simulink model "Imitation_Task_Multi_withSound_withGrid"  (R2015a)
settings: Solver=ode4  SolverMode=MultiTasking  StartTime=0.0  StopTime=inf  FixedStep=BKIN_STEP_TIME  RelTol=1e-3
StartFcn:
  |  warndlg('Dexterit-E models cannot run under simulation. Please compile your model and run it from within Dexterit-E.');set_param(bdroot,'SimulationCommand','stop')
model workspace (MAT data in the model file):
  col_x = 1
  col_y = 2
  RADIUS_VIS = 3
  COLOR_INIT = 4
  START_TARGET_COL = 1
  DELAY_POST_TRIAL_COL = 20
  BKIN_STEP_TIME = 0.00025
  COLOR_MOVE = 5
  START_WAIT_TIME_COL = 2
  CUE_TARGET_COL = 3
  STIM_DUR_COL = 17
  MAX_MOVE_TIME_COL = 18
  HOLD_TIME_COL = 19
  E_START_TRIAL = 2
  E_START_REACHED = 4
  E_MOVED_EARLY = 21
  E_GO_CUE = 9
  E_MOVE_TIMEOUT = 23
  E_HOLDING_STILL = 12
  E_END_TRIAL = 14
  CONTROL_PT1_COL = 8
  CONTROL_PT2_COL = 9
  CONTROL_PT3_COL = 10
  CONTROL_PT4_COL = 11
  STROKE_WIDTH = 6
  K_HAND_VEL = 1
  E_MOVE_ON = 10
  CUE_TYPE_COL = 6
  CUE_VIS_COL = 4
  HAND_VIS_COL = 5
  K_HOLDTIME = 2
  K_ROBOT_RAMP_TIME = 3
  E_ROBOT_RETURN_TO_START = 33
  E_ENABLED_CONTROLLER = 31
  K_TIME_TO_START = 4
  E_RETURN_TO_START = 35
  E_HOLD_POS = 37
  CONTROL_PT5_COL = 12
  CONTROL_PT6_COL = 13
  CONTROL_PT7_COL = 14
  CONTROL_PT8_COL = 15
  CONTROL_PT9_COL = 16
  E_INCREMENTING_TSTEP1 = 6
  E_INCREMENTING_TSTEP2 = 7
  E_INCREMENTING_TSTEP3 = 8
  CONTROL_PT0_COL = 7
  K_TONE_START_FREQUENCY = 5
  K_TONE_START_DURATION = 6
  K_TONE_GO_FREQUENCY = 7
  K_TONE_GO_DURATION = 8
  ENABLE_BKGND_GRID_COL = 21
  BKGND_GRID_TGT_COL = 22
  BKIN_KINEMATIC_FRAME_SIZE = 400
  E_NO_EVENT = 0
libraries: slrtlib x9, Video x7, General x3, KINARM_general x2, KINARM_loads x2, xpcobsoletelib x1, xpcrtudplib x1
CloseFcn:
  | rtwprivate ssgencode ModelCloseRequest b2lab2d
settings Model: ModifiedComment=chris -- Wed Feb 16 09:18:30 2005 -- Version 1.1384  ModifiedHistory=Feb 16/05 - Add error repeat, add offset ramp  ExtModeArmWhenConnect=off  ExtModeLogAll=off  Creator=Chris Grebeldinger  LastModifiedBy=User
settings SolverCC: EnableConcurrentExecution=on  AutoInsertRateTranBlk=on
settings DataIOCC: LimitDataPoints=off  SignalLoggingSaveFormat=ModelDataLogs  SaveOutput=off  SaveTime=off  SignalLoggingName=sigsOut
settings OptimizationCC: BlockReduction=off  BooleanDataType=off  OptimizeBlockIOStorage=off  BufferReuse=off  GlobalBufferReuse=off  ExpressionFolding=off  ExpressionDepthLimit=2147483647  LocalBlockOutputs=off  InitFltsAndDblsToZero=on
settings DebuggingCC: SaveWithParameterizedLinksMsg=none  UnderspecifiedInitializationDetection=Classic  MergeDetectMultiDrivingBlocksExec=none  SignalResolutionControl=TryResolveAllWithWarning  MultiTaskDSMMsg=warning  FcnCallInpInsideContextMsg=UseLocalSettings  StateNameClashWarn=warning  StrictBusMsg=ErrorOnBusTreatedAsVector
settings HardwareCC: ProdIntDivRoundTo=Zero  ProdEndianess=LittleEndian  ProdLongLongMode=on  ProdHWDeviceType=Generic->32-bit x86 compatible  TargetHWDeviceType=32-bit Generic
settings SFSimCC: SimCustomHeaderCode="#include \"stdlib.h\""  SFSimEcho=off  SimParseCustomCode=off
settings RTWCC: SystemTargetFile=slrt.tlc  TemplateMakefile=slrt_default_tmf  Description=Simulink Real-Time  CustomSourceCode="#include \"stdlib.h\""
settings CodeAppCC: MaxIdLength=63
settings SimulinkRealTimeCC: TargetFcnLib=ansi_tfl_tmw.mat  GeneratePreprocessorConditionals=Disable all  xPCisDownloadable=off  xPCisDefaultEnv=off

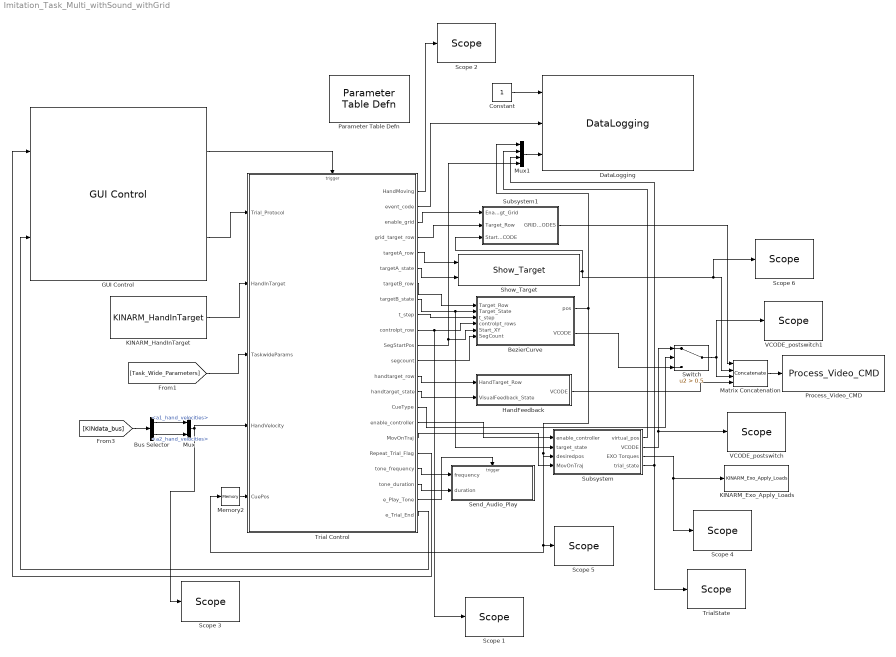
== system Imitation_Task_Multi_withSound_withGrid ==
  BezierCurve : Subsystem
  Bus Selector : BusSelector  OutputSignals=Robot1.a1_hand_velocities,Robot2.a2_hand_velocities
  Constant : Constant
  DataLogging : General/DataLogging  log_event_codes=on  log_analog_inputs=on  show_time_remaining=off
  GUI Control : General/GUI Control  target_type_str=Circle  Target_Type=1  XYcols=[1 2]  Vcols=3  Lcols=4  indices_padding=[0 0 0 0;0 0 0 0]  task_version=1.0  show_repeat_trial_flag=on  target_table_rows=64  load_table_rows=20  tp_table_rows=100
  HandFeedback : Subsystem
  KINARM_Exo_Apply_Loads : KINARM_loads/KINARM_Exo_Apply_Loads  up_duration=200  down_duration=200  max_torque=7  limit_motors=off
  KINARM_HandInTarget : KINARM_general/KINARM_HandInTarget  use_dominant_hand=on  target_type=Circle  num_states=1  attribcol1=[RADIUS_VIS]  attribcol2=[4]  attribcol3=[5]  attribcol4=[6]  attribcol5=[0]
  Matrix Concatenation : Concatenate  NumInputs=4  Mode=Multidimensional array
  Memory2 : Memory  InheritSampleTime=on
  Mux : Mux  Inputs=[2 2]
  Mux1 : Mux
  Parameter Table Defn : General/Parameter Table Defn  ShowInLibBrowser=0
  Process_Video_CMD : Video/Process_Video_CMD  video_delay=50
  Scope 1 : slrtlib/Displays and Logging/Scope   scopeno=2  scopetype=Target  autostart=on  viewmode=Numerical  formatstr='%15.6f'  grid=on  ylimits=[0,0]  nosamples=250  noprepostsamples=0  interleave=1  triggermode=FreeRun  triggersignal=1  trigsignalfromport=off  triggerlevel=0.0  triggerslope=Either  triggerscope=1  triggersample=0  filename=data.dat  mode=Lazy  writesize=512  autorestart=off  dynamicfilemode=off  maxwritefilesize=512*1024^2
  Scope 2 : slrtlib/Displays and Logging/Scope   scopeno=3  scopetype=Target  autostart=on  viewmode=Numerical  formatstr='%15.6f'  grid=on  ylimits=[0,0]  nosamples=250  noprepostsamples=0  interleave=1  triggermode=FreeRun  triggersignal=1  trigsignalfromport=off  triggerlevel=0.0  triggerslope=Either  triggerscope=1  triggersample=0  filename=data.dat  mode=Lazy  writesize=512  autorestart=off  dynamicfilemode=off  maxwritefilesize=512*1024^2
  Scope 3 : slrtlib/Displays and Logging/Scope   scopeno=4  scopetype=Target  autostart=on  viewmode=Numerical  formatstr='%15.6f'  grid=on  ylimits=[0,0]  nosamples=250  noprepostsamples=0  interleave=1  triggermode=FreeRun  triggersignal=1  trigsignalfromport=off  triggerlevel=0.0  triggerslope=Either  triggerscope=1  triggersample=0  filename=data.dat  mode=Lazy  writesize=512  autorestart=off  dynamicfilemode=off  maxwritefilesize=512*1024^2
  Scope 4 : slrtlib/Displays and Logging/Scope   scopeno=5  scopetype=Target  autostart=on  viewmode=Numerical  formatstr='%15.6f'  grid=on  ylimits=[0,0]  nosamples=250  noprepostsamples=0  interleave=1  triggermode=FreeRun  triggersignal=1  trigsignalfromport=off  triggerlevel=0.0  triggerslope=Either  triggerscope=1  triggersample=0  filename=data.dat  mode=Lazy  writesize=512  autorestart=off  dynamicfilemode=off  maxwritefilesize=512*1024^2
  Scope 5 : slrtlib/Displays and Logging/Scope   scopeno=7  scopetype=Target  autostart=on  viewmode=Numerical  formatstr='%15.6f'  grid=on  ylimits=[0,0]  nosamples=250  noprepostsamples=0  interleave=1  triggermode=FreeRun  triggersignal=1  trigsignalfromport=off  triggerlevel=0.0  triggerslope=Either  triggerscope=1  triggersample=0  filename=data.dat  mode=Lazy  writesize=512  autorestart=off  dynamicfilemode=off  maxwritefilesize=512*1024^2
  Scope 6 : slrtlib/Displays and Logging/Scope   scopeno=9  scopetype=Target  autostart=on  viewmode=Numerical  formatstr='%15.6f'  grid=on  ylimits=[0,0]  nosamples=250  noprepostsamples=0  interleave=1  triggermode=FreeRun  triggersignal=1  trigsignalfromport=off  triggerlevel=0.0  triggerslope=Either  triggerscope=1  triggersample=0  filename=data.dat  mode=Lazy  writesize=512  autorestart=off  dynamicfilemode=off  maxwritefilesize=512*1024^2
  Send_Audio_Play : Subsystem  AncestorBlock=General/DataLogging/Network Transfer Subsystem/UDP Send Subsystem  TreatAsAtomicUnit=on
  Show_Target : Video/Show_Target  target_type=Rectangle  num_states=1  attribcol1=[0 COLOR_INIT STROKE_WIDTH RADIUS_VIS RADIUS_VIS 0]  attribcol2=[6 6 0 3 0 0]  attribcol3=[0 0 0 0 0 0]  attribcol4=[0 0 0 0 0 0]  attribcol5=[0 0 24 0 0 0]  stateindices_padding=[0 0 0 0 0;0 0 0 0 0;0 0 0 0 0;0 0 0 0 0;0 0 0 0 0]  source=dialog  opacity=100  target_display=Both subject and operator displays  num_col=6
  Subsystem : Subsystem
  Subsystem1 : Subsystem
  Switch : Switch  Criteria=u2 > Threshold  Threshold=0.5
  Trial Control : Stateflow chart  TreatAsAtomicUnit=on
  TrialState : slrtlib/Displays and Logging/Scope   scopeno=1  scopetype=Target  autostart=on  viewmode=Numerical  formatstr='%15.6f'  grid=on  ylimits=[0,0]  nosamples=250  noprepostsamples=0  interleave=1  triggermode=FreeRun  triggersignal=1  trigsignalfromport=off  triggerlevel=0.0  triggerslope=Either  triggerscope=1  triggersample=0  filename=data.dat  mode=Lazy  writesize=512  autorestart=off  dynamicfilemode=off  maxwritefilesize=512*1024^2
  VCODE_postswitch : slrtlib/Displays and Logging/Scope   scopeno=6  scopetype=Target  autostart=on  viewmode=Numerical  formatstr='%15.6f'  grid=on  ylimits=[0,0]  nosamples=250  noprepostsamples=0  interleave=1  triggermode=FreeRun  triggersignal=1  trigsignalfromport=off  triggerlevel=0.0  triggerslope=Either  triggerscope=1  triggersample=0  filename=data.dat  mode=Lazy  writesize=512  autorestart=off  dynamicfilemode=off  maxwritefilesize=512*1024^2
  VCODE_postswitch1 : slrtlib/Displays and Logging/Scope   scopeno=8  scopetype=Target  autostart=on  viewmode=Numerical  formatstr='%15.6f'  grid=on  ylimits=[0,0]  nosamples=250  noprepostsamples=0  interleave=1  triggermode=FreeRun  triggersignal=1  trigsignalfromport=off  triggerlevel=0.0  triggerslope=Either  triggerscope=1  triggersample=0  filename=data.dat  mode=Lazy  writesize=512  autorestart=off  dynamicfilemode=off  maxwritefilesize=512*1024^2
  wires:
  Trial Control/22(e_Trial_End) -> GUI Control/2
  GUI Control/1 -> Trial Control/Trigger
  Trial Control/6(targetA_state) -> Show_Target/2
  Trial Control/5(targetA_row) -> Show_Target/1
  Matrix Concatenation/1 -> Process_Video_CMD/1
  Trial Control/2(event_code) -> DataLogging/2
  Constant/1 -> DataLogging/1
  GUI Control/2 -> Trial Control/1(Trial_Protocol)
  KINARM_HandInTarget/1 -> Trial Control/2(HandInTarget)
  Trial Control/13(handtarget_row) -> HandFeedback/1(HandTarget_Row)
  Trial Control/14(handtarget_state) -> HandFeedback/2(VisualFeedback_State)
  Show_Target/1 -> Scope 6/1, Matrix Concatenation/2, Subsystem1/3(Start_Tgt_VCODE)
  Trial Control/18(Repeat_Trial_Flag) -> GUI Control/1
  [Task_Wide_Parameters] -> Trial Control/3(TaskwideParams)
  Trial Control/9(t_step) -> BezierCurve/3(t_step)
  Trial Control/7(targetB_row) -> BezierCurve/1(Target_Row)
  Trial Control/10(controlpt_row) -> Scope 1/1, BezierCurve/4(controlpt_rows)
  Trial Control/1(HandMoving) -> Scope 2/1
  Mux/1 -> Trial Control/4(HandVelocity), Scope 3/1
  Bus Selector/1 -> Mux/1  "<a1_hand_velocities>"
  Bus Selector/2 -> Mux/2  "<a2_hand_velocities>"
  Trial Control/15(CueType) -> Switch/2
  Trial Control/16(enable_controller) -> Subsystem/1(enable_controller)
  Trial Control/17(MovOnTraj) -> Subsystem/4(MovOnTraj)
  Mux1/1 -> DataLogging/3
  Subsystem/1(virtual_pos) -> Mux1/2
  Subsystem/3(EXO Torques) -> Scope 4/1, KINARM_Exo_Apply_Loads/1
  BezierCurve/2(VCODE) -> Switch/3
  Subsystem/2(VCODE) -> VCODE_postswitch/1, Switch/1
  Switch/1 -> Matrix Concatenation/3, VCODE_postswitch1/1
  Subsystem/4(trial_state) -> Mux1/3, TrialState/1
  [KINdata_bus] -> Bus Selector/1
  Trial Control/8(targetB_state) -> BezierCurve/2(Target_State), Subsystem/2(target_state)
  Trial Control/11(SegStartPos) -> BezierCurve/5(Start_XY), Mux1/4
  Trial Control/19(tone_frequency) -> Send_Audio_Play/1(frequency)
  Trial Control/20(tone_duration) -> Send_Audio_Play/2(duration)
  Trial Control/21(e_Play_Tone) -> Send_Audio_Play/Trigger
  Trial Control/3(enable_grid) -> Subsystem1/1(Enable_Tgt_Grid)
  Trial Control/4(grid_target_row) -> Subsystem1/2(Target_Row)
  HandFeedback/1(VCODE) -> Matrix Concatenation/4
  Subsystem1/1(GRID_VCODES) -> Matrix Concatenation/1
  BezierCurve/1(pos) -> Memory2/1, Scope 5/1, Subsystem/3(desiredpos), Mux1/1
  Memory2/1 -> Trial Control/5(CuePos)
  Trial Control/12(segcount) -> BezierCurve/6(SegCount)

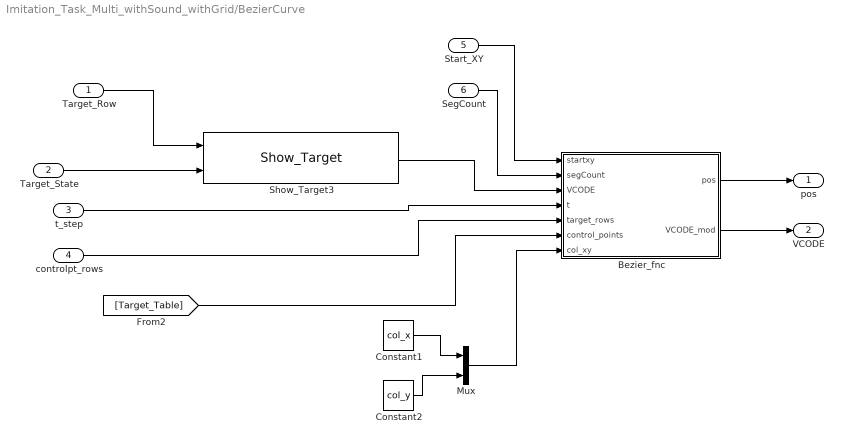
== system Imitation_Task_Multi_withSound_withGrid/BezierCurve ==
  Target_Row : Inport
  Target_State : Inport  Port=2
  t_step : Inport  Port=3
  controlpt_rows : Inport  Port=4
  Start_XY : Inport  Port=5
  SegCount : Inport  Port=6
  Bezier_fnc : MATLAB Function  TreatAsAtomicUnit=on
  Constant1 : Constant  Value=col_x
  Constant2 : Constant  Value=col_y
  Mux : Mux  Inputs=2
  Show_Target3 : Video/Show_Target  target_type=Circle  num_states=1  attribcol1=[COLOR_INIT 0 0 RADIUS_VIS]  attribcol2=[6 6 0 3]  attribcol3=[0 0 0 0]  attribcol4=[0 0 0 0]  attribcol5=[0 0 24 0]  stateindices_padding=[0 0 0 0 0 0 0;0 0 0 0 0 0 0;0 0 0 0 0 0 0;0 0 0 0 0 0 0;0 0 0 0 0 0 0]  source=dialog  opacity=100  target_display=Both subject and operator displays  num_col=4
  pos : Outport
  VCODE : Outport  Port=2
  wires:
  Show_Target3/1 -> Bezier_fnc/3(VCODE)
  Bezier_fnc/2(VCODE_mod) -> VCODE/1
  t_step/1 -> Bezier_fnc/4(t)
  [Target_Table] -> Bezier_fnc/6(control_points)
  controlpt_rows/1 -> Bezier_fnc/5(target_rows)
  Bezier_fnc/1(pos) -> pos/1
  Target_Row/1 -> Show_Target3/1
  Target_State/1 -> Show_Target3/2
  Mux/1 -> Bezier_fnc/7(col_xy)
  Constant1/1 -> Mux/1
  Constant2/1 -> Mux/2
  Start_XY/1 -> Bezier_fnc/1(startxy)
  SegCount/1 -> Bezier_fnc/2(segCount)

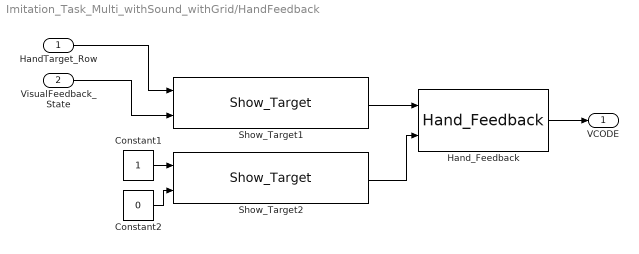
== system Imitation_Task_Multi_withSound_withGrid/HandFeedback ==
  HandTarget_Row : Inport
  VisualFeedback_State : Inport  Port=2
  Constant1 : Constant
  Constant2 : Constant  Value=0
  Hand_Feedback : KINARM_general/Hand_Feedback  feedback_cntl_src=style and status
  Show_Target1 : Video/Show_Target  target_type=Circle  num_states=2  attribcol1=[COLOR_INIT 0 0 RADIUS_VIS]  attribcol2=[COLOR_MOVE 0 0 RADIUS_VIS]  attribcol3=[0 0 0 0]  attribcol4=[0 0 0 0]  attribcol5=[0 0 24 0]  stateindices_padding=[0 0 0 0 0 0 0;0 0 0 0 0 0 0;0 0 0 0 0 0 0;0 0 0 0 0 0 0;0 0 0 0 0 0 0]  source=dialog  opacity=100  target_display=Both subject and operator displays  num_col=4
  Show_Target2 : Video/Show_Target  target_type=Circle  num_states=2  attribcol1=[COLOR_INIT 0 0 RADIUS_VIS]  attribcol2=[COLOR_MOVE 0 0 RADIUS_VIS]  attribcol3=[0 0 0 0]  attribcol4=[0 0 0 0]  attribcol5=[0 0 24 0]  stateindices_padding=[0 0 0 0 0 0 0;0 0 0 0 0 0 0;0 0 0 0 0 0 0;0 0 0 0 0 0 0;0 0 0 0 0 0 0]  source=dialog  opacity=100  target_display=Both subject and operator displays  num_col=4
  VCODE : Outport
  wires:
  Show_Target1/1 -> Hand_Feedback/1
  HandTarget_Row/1 -> Show_Target1/1
  VisualFeedback_State/1 -> Show_Target1/2
  Constant1/1 -> Show_Target2/1
  Constant2/1 -> Show_Target2/2
  Show_Target2/1 -> Hand_Feedback/2
  Hand_Feedback/1 -> VCODE/1

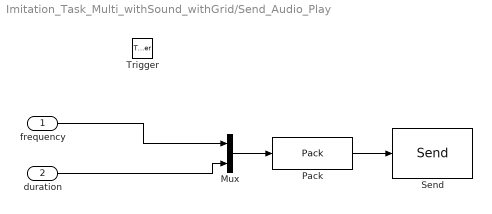
== system Imitation_Task_Multi_withSound_withGrid/Send_Audio_Play ==
  frequency : Inport
  duration : Inport  Port=2
  Trigger : TriggerPort  TriggerType=either
  Mux : Mux  Inputs=2
  Pack : xpcobsoletelib/Utilities/Pack   datatypes={'int32'}  byteAlign=1
  Send : xpcrtudplib/Legacy UDP/Send   ipAddress=255.255.255.255  ipPort=25255  localPort=-1  vblLen=off  sampletime=-1
  wires:
  frequency/1 -> Mux/1
  duration/1 -> Mux/2
  Mux/1 -> Pack/1
  Pack/1 -> Send/1

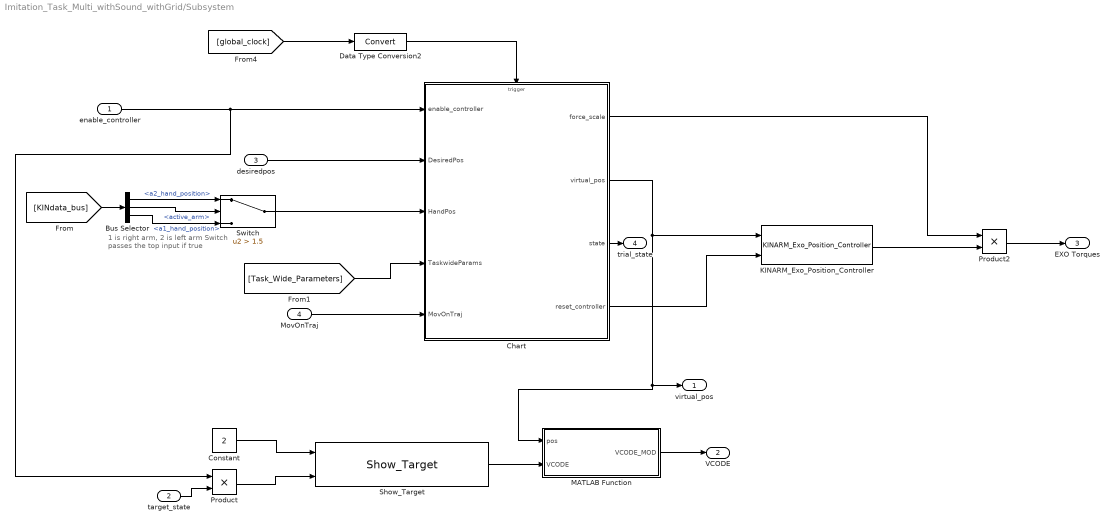
== system Imitation_Task_Multi_withSound_withGrid/Subsystem ==
  note: 1 is right arm, 2 is left arm
      | Switch passes the top input if true
  enable_controller : Inport
  target_state : Inport  Port=2
  desiredpos : Inport  Port=3
  MovOnTraj : Inport  Port=4
  Bus Selector : BusSelector  OutputSignals=Robot2.a2_hand_position,KINDataGeneral.active_arm,Robot1.a1_hand_position
  Chart : Stateflow chart  TreatAsAtomicUnit=on
  Constant : Constant  Value=2
  Data Type Conversion2 : DataTypeConversion
  KINARM_Exo_Position_Controller : KINARM_loads/KINARM_Exo_Position_Controller  use_dom_hand=on  KINARM_Type=Human  inertias_for_FF=KINARM robot & arm troughs & subject  angles_or_XY=End-point (global x/y)  sample_time=0.001
  MATLAB Function : MATLAB Function  TreatAsAtomicUnit=on
  Product : Product
  Product2 : Product
  Show_Target : Video/Show_Target  target_type=Circle  num_states=1  attribcol1=[COLOR_INIT 0 0 RADIUS_VIS]  attribcol2=[6 6 0 3]  attribcol3=[0 0 0 0]  attribcol4=[0 0 0 0]  attribcol5=[0 0 24 0]  stateindices_padding=[0 0 0 0 0 0 0;0 0 0 0 0 0 0;0 0 0 0 0 0 0;0 0 0 0 0 0 0;0 0 0 0 0 0 0]  source=dialog  opacity=100  target_display=Both subject and operator displays  num_col=4
  Switch : Switch  Criteria=u2 > Threshold  Threshold=1.5
  virtual_pos : Outport
  VCODE : Outport  Port=2
  EXO Torques : Outport  Port=3
  trial_state : Outport  Port=4
  wires:
  [KINdata_bus] -> Bus Selector/1
  Bus Selector/2 -> Switch/2  "<active_arm>"
  [Task_Wide_Parameters] -> Chart/4(TaskwideParams)
  [global_clock] -> Data Type Conversion2/1
  Data Type Conversion2/1 -> Chart/Trigger
  Chart/2(virtual_pos) -> MATLAB Function/1(pos), virtual_pos/1, KINARM_Exo_Position_Controller/1
  MovOnTraj/1 -> Chart/5(MovOnTraj)
  Switch/1 -> Chart/3(HandPos)
  desiredpos/1 -> Chart/2(DesiredPos)
  Constant/1 -> Show_Target/1
  Show_Target/1 -> MATLAB Function/2(VCODE)
  MATLAB Function/1(VCODE_MOD) -> VCODE/1
  KINARM_Exo_Position_Controller/1 -> Product2/2
  Product2/1 -> EXO Torques/1
  Chart/1(force_scale) -> Product2/1
  Chart/4(reset_controller) -> KINARM_Exo_Position_Controller/2
  Bus Selector/1 -> Switch/1  "<a2_hand_position>"
  Bus Selector/3 -> Switch/3  "<a1_hand_position>"
  Chart/3(state) -> trial_state/1
  enable_controller/1 -> Product/1, Chart/1(enable_controller)
  Product/1 -> Show_Target/2
  target_state/1 -> Product/2

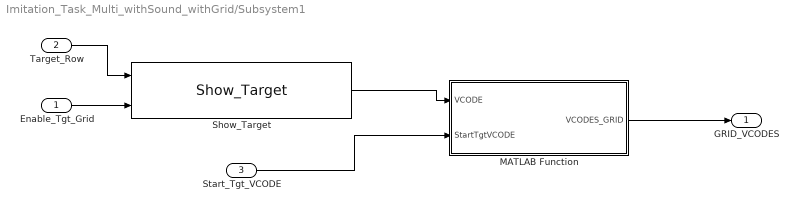
== system Imitation_Task_Multi_withSound_withGrid/Subsystem1 ==
  Enable_Tgt_Grid : Inport
  Target_Row : Inport  Port=2
  Start_Tgt_VCODE : Inport  Port=3
  MATLAB Function : MATLAB Function  TreatAsAtomicUnit=on
  Show_Target : Video/Show_Target  target_type=Circle  num_states=1  attribcol1=[COLOR_INIT 0 0 RADIUS_VIS]  attribcol2=[6 6 0 3]  attribcol3=[0 0 0 0]  attribcol4=[0 0 0 0]  attribcol5=[0 0 24 0]  stateindices_padding=[0 0 0 0 0 0 0;0 0 0 0 0 0 0;0 0 0 0 0 0 0;0 0 0 0 0 0 0;0 0 0 0 0 0 0]  source=dialog  opacity=100  target_display=Both subject and operator displays  num_col=4
  GRID_VCODES : Outport
  wires:
  Target_Row/1 -> Show_Target/1
  Enable_Tgt_Grid/1 -> Show_Target/2
  MATLAB Function/1(VCODES_GRID) -> GRID_VCODES/1
  Show_Target/1 -> MATLAB Function/1(VCODE)
  Start_Tgt_VCODE/1 -> MATLAB Function/2(StartTgtVCODE)

== stateflow chart Imitation_Task_Multi_withSound_withGrid/Subsystem/Chart ==
  state EnableState/
    state AutoMoveToPos/
      //smoothly creates a trajectory to get the hand to a point eventually
      state MovingToDesiredXY/
        tickCount = TaskwideParams[K_TIME_TO_START];
        state = 11;
        tick = 0;
        during:
        on e_clk: tick++;
        // the trajectory velocity will have a bell shaped profile
        trajectory_shape = tick/tickCount-sin(2*pi*tick/tickCount)/(2*pi);
        virtual_pos[1] = StartPos[1] + (TgtPos[1] - StartPos[1]) * trajectory_shape;
        virtual_pos[2] = StartPos[2] + (TgtPos[2] - StartPos[2]) * trajectory_shape;
      state GetDesiredXY/
        //grab the current desired pos in case it changes
        TgtPos[1] = DesiredPos[1];
        TgtPos[2] = DesiredPos[2];
        StartPos[1] = HandPos[1];
        StartPos[2] = HandPos[2];
        updatepos = 0;
        state = 10;
      state HoldAtDesiredXY/
        //pause until something changes
        state = 12;
        updatepos = 0;
        during:
        on e_clk: updatepos = ( (abs(TgtPos[1]-DesiredPos[1]) > 0.01) || (abs(TgtPos[2]-DesiredPos[2]) > 0.01) )
      GetDesiredXY -> MovingToDesiredXY : after(1, e_clk)
      HoldAtDesiredXY -> GetDesiredXY : [updatepos == 1 && MovOnTraj == 0]
      MovingToDesiredXY -> HoldAtDesiredXY : after(tickCount, e_clk)/
    state MoveAlongTraj/
      //take a step along a trajectory specified externally
      state GetDesiredXY_Traj/
        TgtPos[1] = DesiredPos[1];
        TgtPos[2] = DesiredPos[2];
        StartPos[1] = HandPos[1];
        StartPos[2] = HandPos[2];
        state = 21;
        //movIsSafe = ( (abs(TgtPos[1]-HandPos[1]) < 0.02) || (abs(TgtPos[2]-HandPos[2]) < 0.02) );
        movIsSafe = 1;
      state MovAlongTraj/
        state = 22;
        virtual_pos[1] = DesiredPos[1];
        virtual_pos[2] = DesiredPos[2];
      GetDesiredXY_Traj -> MovAlongTraj [order 2] : [movIsSafe == 1]
      MovAlongTraj -> GetDesiredXY_Traj
    (junction 15) -> GetDesiredXY [order 1] : [MovOnTraj == 0]
    (junction 15) -> GetDesiredXY_Traj [order 2] : [MovOnTraj == 1]
    MoveAlongTraj -> GetDesiredXY : [MovOnTraj == 0]
    GetDesiredXY_Traj -> GetDesiredXY [order 1] : [movIsSafe == 0]
    AutoMoveToPos -> GetDesiredXY_Traj : [MovOnTraj == 1]
  state Init/
    ramp_time = TaskwideParams[K_ROBOT_RAMP_TIME];
    scale_increment = 1/ramp_time;
    force_scale = 0;
    state = 1;
    during:
    CurHandPos[1] = HandPos[1];
    CurHandPos[2] = HandPos[2];
  state RampUp/
    //ramp up the force scale to 1
    CurHandPos[1] = HandPos[1];
    CurHandPos[2] = HandPos[2];
    virtual_pos[1] = HandPos[1];
    virtual_pos[2] = HandPos[2];
    state = 2;
    force_scale = 0;
    during:
    on e_clk: force_scale += scale_increment;
  state ResetController/
    reset_controller;
  state RampDown/
    //ramp down the force scale to 1
    CurHandPos[1] = HandPos[1];
    CurHandPos[2] = HandPos[2];
    virtual_pos[1] = CurHandPos[1];
    virtual_pos[2] = CurHandPos[2];
    state = 30
    during:
    on e_clk: force_scale -= scale_increment;
  (default) -> Init
  Init -> ResetController : //if controller becomes enabled
      | [enable_controller == 1]/
      | force_scale = 0;
  ResetController -> RampUp
  RampUp -> (junction 15) [order 2] : [force_scale >= 1]/
      | force_scale = 1;
  RampDown -> Init [order 2] : [force_scale <0]/
      | force_scale = 0;
  RampDown -> RampUp [order 1] : [enable_controller == 1]
      | //if the controller is enabled
  RampUp -> RampDown [order 1] : [enable_controller == 0]
      | //if the controller gets shut off
  EnableState -> RampDown : [enable_controller == 0]
  data: enable_controller input boolean; DesiredPos input; HandPos input; TaskwideParams input; force_scale output double; virtual_pos output double size=2; tickCount local double; StartPos local double size=2; TgtPos local double size=2; updatepos local boolean; MovOnTraj input double; CurHandPos local double size=2; ramp_time local double; scale_increment local double; tick local double; trajectory_shape local double; movIsSafe local boolean; pi constant double =3.14159265358979; state output double
  events: e_clk input EITHER_EDGE_EVENT; reset_controller output EITHER_EDGE_EVENT

== stateflow chart Imitation_Task_Multi_withSound_withGrid/Trial Control ==
  state MainTrial
    state ShowStartTarget/
      // Turn on start target and wait for a specified time or until the hand is in the target.
      event_code = E_START_TRIAL;
      targetA_row = Trial_Protocol[START_TARGET_COL];
      targetA_state = 1;
      enable_controller = 0;
      SegStartPos[1] = 0;
      SegStartPos[2] = 0;
      enable_grid = Trial_Protocol[ENABLE_BKGND_GRID_COL];
      grid_target_row = Trial_Protocol[BKGND_GRID_TGT_COL];
    state HoldInStart/
      // Log an event that target was reached and then wait for a specified time.
      event_code = E_START_REACHED;
      tickCount = Trial_Protocol[START_WAIT_TIME_COL] ;
      t_step = 0;
      CueType = Trial_Protocol[CUE_TYPE_COL];
      targetB_row = Trial_Protocol[CUE_TARGET_COL];
      controlpt_row[1] = Trial_Protocol[START_TARGET_COL];
      controlpt_row[2] = -1;
      controlpt_row[3] = -1;
      controlpt_row[4] = -1;
      t_step = 0;
      SegStartPos[1] = 0;
      SegStartPos[2] = 0;
      segcount = 0;
    state ProprioceptiveCue/
      state RampOnController/
        targetB_row = Trial_Protocol[CUE_TARGET_COL];
        targetB_state = Trial_Protocol[CUE_VIS_COL];
        SegStartPos[1] = 0.0;
        SegStartPos[2] = 0.0;
        segcount = 0;
        controlpt_row[1] = Trial_Protocol[START_TARGET_COL];
        controlpt_row[2] = -1;
        controlpt_row[3] = -1;
        controlpt_row[4] = -1;
        t_step = 0;
        enable_controller = 1;
        event_code = E_ENABLED_CONTROLLER;
        MovOnTraj = 0;
      state MoveToCP1/
        //shift the hand into control point 1, which may nudge the hand slightly to center it
        event_code = E_RETURN_TO_START;
        tickCount = TaskwideParams[K_TIME_TO_START];
        MovOnTraj = 0;
        t_step = 0;
      state ImitationStimCounterP1/
        // The hand is in the start position so start incrementing t_step
        event_code = E_INCREMENTING_TSTEP1;
        targetB_row = Trial_Protocol[CUE_TARGET_COL];
        targetB_state = Trial_Protocol[CUE_VIS_COL];
        handtarget_state = Trial_Protocol[HAND_VIS_COL];
        SegStartPos[1] = CuePos[1];
        SegStartPos[2] = CuePos[2];
        segcount = 1;
        controlpt_row[1] = Trial_Protocol[CONTROL_PT0_COL];
        controlpt_row[2] = Trial_Protocol[CONTROL_PT1_COL];
        controlpt_row[3] = Trial_Protocol[CONTROL_PT2_COL];
        controlpt_row[4] = Trial_Protocol[CONTROL_PT3_COL];
        MovOnTraj = 1;
        [last_control_pt1,t_step] = findLastCtlPt(controlpt_row[1],controlpt_row[2],controlpt_row[3],controlpt_row[4]);
        during:
        on e_clk: t_step = t_step + (1/ (Trial_Protocol[STIM_DUR_COL]/1000 * 1000)); //increment t_step on each clock cycle
      state ImitationStimCounterP2/
        // The hand is in the start position so start incrementing t_step
        event_code = E_INCREMENTING_TSTEP2;
        SegStartPos[1] = CuePos[1];
        SegStartPos[2] = CuePos[2];
        segcount = 2;
        controlpt_row[1] = Trial_Protocol[CONTROL_PT0_COL];
        controlpt_row[2] = Trial_Protocol[CONTROL_PT4_COL];
        controlpt_row[3] = Trial_Protocol[CONTROL_PT5_COL];
        controlpt_row[4] = Trial_Protocol[CONTROL_PT6_COL];
        MovOnTraj = 1;
        t_step = 0;
        [last_control_pt2,t_step] = findLastCtlPt(controlpt_row[1],controlpt_row[2],controlpt_row[3],controlpt_row[4]);
        //if (indlcp <= 1.01)
        //	t_step = 1;
        //end
        during:
        on e_clk: t_step = t_step + (1/ (Trial_Protocol[STIM_DUR_COL]/1000 * 1000)); //increment t_step on each clock cycle
      state ImitationStimCounterP3/
        // The hand is in the start position so start incrementing t_step
        event_code = E_INCREMENTING_TSTEP3;
        SegStartPos[1] = CuePos[1];
        SegStartPos[2] = CuePos[2];
        segcount = 3;
        controlpt_row[1] = Trial_Protocol[CONTROL_PT0_COL];
        controlpt_row[2] = Trial_Protocol[CONTROL_PT7_COL];
        controlpt_row[3] = Trial_Protocol[CONTROL_PT8_COL];
        controlpt_row[4] = Trial_Protocol[CONTROL_PT9_COL];
        MovOnTraj = 1;
        t_step = 0;
        [last_control_pt3,t_step] = findLastCtlPt(controlpt_row[1],controlpt_row[2],controlpt_row[3],controlpt_row[4]);
        //if (indlcp <= 1.01)
        //	t_step = 1;
        //end
        during:
        on e_clk: t_step = t_step + (1/ (Trial_Protocol[STIM_DUR_COL]/1000 * 1000)); //increment t_step on each clock cycle
      state CueEndHoldP/
        //pause at the end of the cue
        event_code = E_HOLD_POS;
        //tickCount = TaskwideParams[K_HOLDTIME];
        MovOnTraj = 1;
        tone_frequency=TaskwideParams[K_TONE_START_FREQUENCY];
        tone_duration=TaskwideParams[K_TONE_START_DURATION];
        e_Play_Tone;
        tickCount = 500;
        //controlpt_row[1] = Trial_Protocol[last_control_pt3];
        //controlpt_row[2] = Trial_Protocol[last_control_pt3];
        //controlpt_row[3] = -1;
        //controlpt_row[4] = -1;
        t_step = 1;
      state CueEndHoldP1/
        //pause at the end of the cue
        tickCount = TaskwideParams[K_HOLDTIME];
        MovOnTraj = 1;
        //play the tone twice to signal the end of the cue period
        e_Play_Tone;
        t_step = 1;
      state ReturnToStartP/
        //pause at the end of the cue
        event_code = E_ROBOT_RETURN_TO_START;
        //targetB_row = Trial_Protocol[CUE_TARGET_COL];
        SegStartPos[1] = 0.0;
        SegStartPos[2] = 0.0;
        segcount = 0;
        controlpt_row[1] = Trial_Protocol[START_TARGET_COL];
        controlpt_row[2] = -1;
        controlpt_row[3] = -1;
        controlpt_row[4] = -1;
        MovOnTraj = 0;
        t_step = 0;
        tickCount = TaskwideParams[K_TIME_TO_START];
        during:
        //on e_clk:  t_step = t_step - (1/ (Trial_Protocol[STIM_DUR_COL]/1000 * 1000));
      state CueGoHoldP/
        //pause at the end of the movement return
        tickCount = ramp_time;
        handtarget_state = 1;
        enable_controller = 0;
      RampOnController -> MoveToCP1 : after(ramp_time, e_clk)
      MoveToCP1 -> ImitationStimCounterP1 : [after(tickCount,e_clk)]/
          | t_step = 0;
          | tone_frequency=TaskwideParams[K_TONE_START_FREQUENCY];
          | tone_duration=TaskwideParams[K_TONE_START_DURATION];
          | e_Play_Tone;
          | //HandInTarget[Trial_Protocol[CONTROL_PT1_COL]] &&
      ImitationStimCounterP1 -> ImitationStimCounterP2 : [(t_step >= 1)]/
          | t_step = 1;
          | //SegStartPos[1] = CuePos[1];
          | //SegStartPos[2] = CuePos[2];
          | //&& HandInTarget[Trial_Protocol[last_control_pt]] == 1
          | //if proprioceptively cued, pause
          | //then return hand to start position
      ImitationStimCounterP2 -> ImitationStimCounterP3 : [(t_step >= 1)]/
          | t_step = 1;
          | //SegStartPos[1] = CuePos[1];
          | //SegStartPos[2] = CuePos[2];
          | //&& HandInTarget[Trial_Protocol[last_control_pt2]] == 1
          | //if proprioceptively cued, pause
          | //then return hand to start position
      ImitationStimCounterP3 -> CueEndHoldP : [(t_step >= 1)]/
          | t_step = 1;
          | //&& HandInTarget[Trial_Protocol[last_control_pt3]] == 1
          | //if proprioceptively cued, pause
          | //then return hand to start position
      CueEndHoldP -> CueEndHoldP1 : after(tickCount,e_clk)
      CueEndHoldP1 -> ReturnToStartP : after(tickCount,e_clk)
      ReturnToStartP -> CueGoHoldP : after(tickCount,e_clk)
          | //when the hand returns to the start position
    state VisualCue/
      state ImitationStimCounterV1/
        // The hand has stayed in the start position so start incrementing t_step
        event_code = E_INCREMENTING_TSTEP1;
        CueType = Trial_Protocol[CUE_TYPE_COL];
        SegStartPos[1] = CuePos[1];
        SegStartPos[2] = CuePos[2];
        segcount = 1;
        targetB_state = 1;
        targetB_row = Trial_Protocol[CUE_TARGET_COL];
        handtarget_state = Trial_Protocol[HAND_VIS_COL];
        controlpt_row[1] = Trial_Protocol[CONTROL_PT0_COL];
        controlpt_row[2] = Trial_Protocol[CONTROL_PT1_COL];
        controlpt_row[3] = Trial_Protocol[CONTROL_PT2_COL];
        controlpt_row[4] = Trial_Protocol[CONTROL_PT3_COL];
        t_step = 0;
        [last_control_pt1,t_step] = findLastCtlPt(controlpt_row[1],controlpt_row[2],controlpt_row[3],controlpt_row[4]);
        tone_frequency=TaskwideParams[K_TONE_START_FREQUENCY];
        tone_duration=TaskwideParams[K_TONE_START_DURATION];
        e_Play_Tone;
        during:
        on e_clk: t_step = t_step + (1/ (Trial_Protocol[STIM_DUR_COL]/1000 * 1000)); //increment t_step on each clock cycle
      state ImitationStimCounterV2/
        // The hand has stayed in the start position so start incrementing t_step
        event_code = E_INCREMENTING_TSTEP2;
        SegStartPos[1] = CuePos[1];
        SegStartPos[2] = CuePos[2];
        segcount = 2;
        controlpt_row[1] = Trial_Protocol[CONTROL_PT0_COL];
        controlpt_row[2] = Trial_Protocol[CONTROL_PT4_COL];
        controlpt_row[3] = Trial_Protocol[CONTROL_PT5_COL];
        controlpt_row[4] = Trial_Protocol[CONTROL_PT6_COL];
        t_step = 0;
        [last_control_pt2,t_step] = findLastCtlPt(controlpt_row[1],controlpt_row[2],controlpt_row[3],controlpt_row[4]);
        during:
        on e_clk: t_step = t_step + (1/ (Trial_Protocol[STIM_DUR_COL]/1000 * 1000)); //increment t_step on each clock cycle
      state HandMovedEarlyV/
        event_code = E_MOVED_EARLY;
        Repeat_Trial_Flag = 1;
      state ImitationStimCounterV3/
        // The hand has stayed in the start position so start incrementing t_step
        event_code = E_INCREMENTING_TSTEP3;
        SegStartPos[1] = CuePos[1];
        SegStartPos[2] = CuePos[2];
        segcount = 3;
        controlpt_row[1] = Trial_Protocol[CONTROL_PT0_COL];
        controlpt_row[2] = Trial_Protocol[CONTROL_PT7_COL];
        controlpt_row[3] = Trial_Protocol[CONTROL_PT8_COL];
        controlpt_row[4] = Trial_Protocol[CONTROL_PT9_COL];
        t_step = 0;
        [last_control_pt3,t_step] = findLastCtlPt(controlpt_row[1],controlpt_row[2],controlpt_row[3],controlpt_row[4]);
        during:
        on e_clk: t_step = t_step + (1/ (Trial_Protocol[STIM_DUR_COL]/1000 * 1000)); //increment t_step on each clock cycle
      state CueEndHoldV/
        //pause at the end of the cue
        tone_frequency=TaskwideParams[K_TONE_START_FREQUENCY];
        tone_duration=TaskwideParams[K_TONE_START_DURATION];
        e_Play_Tone;
        tickCount = 500;
      state CueEndHoldV1/
        //pause at the end of the cue
        tickCount = TaskwideParams[K_HOLDTIME];
        //play the tone twice to signal the end of the cue period
        e_Play_Tone;
      ImitationStimCounterV1 -> HandMovedEarlyV [order 2] : //If visually-cued and hand leaves target
          | [HandInTarget[targetA_row]==0]
      ImitationStimCounterV1 -> ImitationStimCounterV2 [order 1] : [after(1,e_clk) && t_step >= 1]/
          | t_step = 1;
          | //SegStartPos[1] = CuePos[1];
          | //SegStartPos[2] = CuePos[2];
      ImitationStimCounterV2 -> HandMovedEarlyV [order 1] : //If visually-cued and hand leaves target
          | [HandInTarget[targetA_row]==0]
      ImitationStimCounterV3 -> HandMovedEarlyV [order 1] : //If visually-cued and hand leaves target
          | [HandInTarget[targetA_row]==0]
      ImitationStimCounterV2 -> ImitationStimCounterV3 [order 2] : [after(1,e_clk) && t_step >= 1]/
          | t_step = 1;
          | //SegStartPos[1] = CuePos[1];
          | //SegStartPos[2] = CuePos[2];
      ImitationStimCounterV3 -> CueEndHoldV [order 2] : [after(1,e_clk) && t_step >= 1]/
          | t_step = 1;
      CueEndHoldV -> CueEndHoldV1 : after(tickCount,e_clk)
    state GoCue/
      event_code = E_GO_CUE;
      targetA_state = 0;
      targetB_state = 0;
      handtarget_state = 2;
      tone_frequency=TaskwideParams[K_TONE_GO_FREQUENCY];
      tone_duration=TaskwideParams[K_TONE_GO_DURATION];
      e_Play_Tone;
      tickCount = Trial_Protocol[MAX_MOVE_TIME_COL];
      during:
      HandMoving[1] = abs(HandVelocity[1]) >= (TaskwideParams[K_HAND_VEL]*2);
      HandMoving[2] = abs(HandVelocity[2]) >= (TaskwideParams[K_HAND_VEL]*2);
      HandMoving[3] = abs(HandVelocity[3]) >= (TaskwideParams[K_HAND_VEL]*2);
      HandMoving[4] = abs(HandVelocity[4]) >= (TaskwideParams[K_HAND_VEL]*2);
    state MovingState/
      // If movement started, check arm velocity to detect movement offset
      event_code = E_MOVE_ON;
      handtarget_state = handtarget_state*Trial_Protocol[HAND_VIS_COL];
      //if (Trial_Protocol[HAND_VIS_COL]==0)
      //	handtarget_state = 0;
      //end
      during:
      HandMoving[1] = abs(HandVelocity[1]) >= TaskwideParams[K_HAND_VEL];
      HandMoving[2] = abs(HandVelocity[2]) >= TaskwideParams[K_HAND_VEL];
      HandMoving[3] = abs(HandVelocity[3]) >= TaskwideParams[K_HAND_VEL];
      HandMoving[4] = abs(HandVelocity[4]) >= TaskwideParams[K_HAND_VEL];
      if (HandMoving[1] || HandMoving[2] || HandMoving[3] || HandMoving[4] && stateiter>1000)
      movVelThreshHit = 1;
      end
      on e_clk: stateiter = stateiter+1;
    state MovementTimeout/
      event_code = E_MOVE_TIMEOUT;
      //handtarget_state = 0;
    state HandStill/
      // check if the hand velocity is still below threshold
      event_code = E_HOLDING_STILL;
      tickCount = Trial_Protocol[HOLD_TIME_COL];
      during:
      HandMoving[1] = abs(HandVelocity[1]) >= TaskwideParams[K_HAND_VEL];
      HandMoving[2] = abs(HandVelocity[2]) >= TaskwideParams[K_HAND_VEL];
      HandMoving[3] = abs(HandVelocity[3]) >= TaskwideParams[K_HAND_VEL];
      HandMoving[4] = abs(HandVelocity[4]) >= TaskwideParams[K_HAND_VEL];
      on e_clk: stateiter = stateiter+1;
    state EndOfTrial/
      // Turn off the target, set the post-trial delay
      event_code = E_END_TRIAL;
      targetA_state = 0;
      handtarget_state = 0;
      tickCount = Trial_Protocol[DELAY_POST_TRIAL_COL];
    ShowStartTarget -> HoldInStart : // is the hand in the target?
        | [HandInTarget[targetA_row] == 1]
    HoldInStart -> ShowStartTarget [order 2] : [HandInTarget[targetA_row]==0]
    HoldInStart -> (junction 114) [order 1] : after(tickCount,e_clk)
    (junction 114) -> ImitationStimCounterV1 [order 2] : // has a a specified period of
        | // time occured?
        | [CueType == 0]
    (junction 114) -> RampOnController [order 1] : // has a a specified period of
        | // time occured?
        | [CueType == 1]
    HandMovedEarlyV -> EndOfTrial
    CueGoHoldP -> GoCue : after(tickCount,e_clk)
    CueEndHoldV1 -> GoCue : after(tickCount,e_clk)
    GoCue -> MovementTimeout [order 1] : after(tickCount,e_clk)
    GoCue -> MovingState [order 2] : [HandInTarget[targetA_row]==0 || (HandMoving[1] || HandMoving[2] || HandMoving[3] || HandMoving[4])]/
        | //if hand left start position or started moving
        | movVelThreshHit = 0;
        | stateiter = 0;
    MovingState -> MovementTimeout [order 2] : //check from time first entered the state
        | [stateiter >= Trial_Protocol[MAX_MOVE_TIME_COL]]
    MovementTimeout -> EndOfTrial
    MovingState -> HandStill [order 1] : [movVelThreshHit && !HandMoving[1] && !HandMoving[2] && !HandMoving[3] && !HandMoving[4]]
    HandStill -> MovingState [order 2] : [HandMoving[1] || HandMoving[2] || HandMoving[3] || HandMoving[4]]
    HandStill -> EndOfTrial [order 1] : after(tickCount,e_clk)
  state Initialize/
    //Initialization state
    targetA_state = 0;
    targetB_state = 0;
    handtarget_state = 1;
    handtarget_row = 3;
    Repeat_Trial_Flag = 0;
    ramp_time = TaskwideParams[K_ROBOT_RAMP_TIME];
    enable_controller = 0;
    enable_grid = 0;
    segcount = -1
  state Inter_Trial_State/
    // Turn off target, reset the event code, and send the
    //e_Trial_End Stateflow event to indicate that the trial is over.
    event_code = 0;
    targetA_state = 0;
    targetB_state = 0;
    handtarget_state = 1;
    Repeat_Trial_Flag = 0;
    enable_grid = 0;
    segcount = -1;
    e_Trial_End;
  state RobotRampDown/
    enable_controller = 0;
  note: ?
  Initialize -> ShowStartTarget
  (default) -> Initialize
  Inter_Trial_State -> ShowStartTarget : // has a a specified period of
      | // time occured?
      | after(tickCount, e_clk)
  (junction 116) -> Inter_Trial_State [order 1]
  MainTrial -> (junction 116) : e_ExitTrialNow/
      | tickCount = 1;
      | // e_ExitTrialNow event occurs if the
      | // Dex pause is pressed by the operator
  (junction 116) -> RobotRampDown [order 2] : [controller_on == 1]
  EndOfTrial -> Inter_Trial_State : after(tickCount,e_clk)
  RobotRampDown -> Inter_Trial_State : after(ramp_time,e_clk)
  data: cp1 function_input double; cp2 function_input double; cp3 function_input double; cp4 function_input double; lcp function_output double; t function_output double; HandMoving output boolean size=4; event_code output uint16 [0..] =0; enable_grid output double; grid_target_row output double; targetA_row output [1..32]; targetA_state output double; tickCount local double; Trial_Protocol input double; HandInTarget input double; TaskwideParams input double; HandVelocity input double; targetB_row output double; targetB_state output double; t_step output double; controlpt_row output double size=4; SegStartPos output double size=2; segcount output double; handtarget_row output double; handtarget_state output double; movVelThreshHit local boolean; stateiter local double; CueType output double; ramp_time local double; enable_controller output boolean; MovOnTraj output double; Repeat_Trial_Flag output double; last_control_pt1 local double =0; last_control_pt2 local double =0; last_control_pt3 local double =0; CuePos input double size=2; tone_frequency output int32; tone_duration output int32
  data targetA_row settings: description=index of the row currently being used in the TargetTable
  events: e_Play_Tone output EITHER_EDGE_EVENT; e_clk input RISING_EDGE_EVENT; e_ExitTrialNow input EITHER_EDGE_EVENT; e_Trial_End output EITHER_EDGE_EVENT
  function [lcp,t]  = findLastCtlPt(cp1,cp2,cp3,cp4):
    | function [lcp,t]  = findLastCtlPt(cp1,cp2,cp3,cp4)
    | 
    | %find the index to the last control point in the TP table
    | 
    | 
    | lcp = 0;
    | indlcp = 0;
    | 
    | if (cp4 > 0)
    | 	lcp = cp4;
    |     indlcp = 4;
    |     t = 0;
    | elseif (cp3 > 0)
    | 	lcp = cp3;
    |     indlcp = 3;
    |     t = 0;
    | elseif (cp2 > 0)
    | 	lcp = cp2;
    |     indlcp = 2;
    |     t = 0;
    | else
    | 	lcp = cp1;
    |     indlcp = 1;
    |     t = 1;
    | end

== matlab function Imitation_Task_Multi_withSound_withGrid/BezierCurve/Bezier_fnc ==
  data: startxy input; segCount input; pos output; VCODE input; VCODE_mod output; t input; target_rows input; control_points input; col_xy input
function [pos,VCODE_mod] = fcn(startxy,segCount,VCODE,t,target_rows,control_points,col_xy)
%#codegen

VCODE_mod = VCODE;

%startxy is the absolute starting point for the segment

%find all the nonzero (valid) control points
target_rows = target_rows(target_rows>0);

offsetX = 0;
offsetY = 0;
if segCount > 0 %(all(abs(startxy) > 0.01))
    
    %this is the starting (x,y) position for this segment in cm, i.e., "(0,0)"
    %the difference between this and the absolute segment starting position
    %gives us the offset
    startX = control_points(target_rows(1),col_xy(1));
    startY = control_points(target_rows(1),col_xy(2));
    
    offsetX = startxy(1)-(startX/100);
    offsetY = startxy(2)-(startY/100);
end



%clip t just in case!
if t < 0
    t = 0;
elseif t > 1;
    t = 1;
end

%t_hat = [0:0.001:1];

%reshape t from purely linear to sigmoidal, to nicely shape the speed
%k = 20;
%t = 1/(1+exp(-k*(t-0.5)));

t = t-sin(2*pi*t)/(2*pi);  %use the bell-shaped velocity profile from the trajectory controller


%we will fill in the Bezier curve code here

if (length(target_rows) == 3)
    
%     %reshape t from purely linear to some nicely shaped speed following the
%     %2/3 power law?
%     x = ((1-t_hat).^2)*control_points(target_rows(1),col_xy(1)) + 2*(t_hat.*(1-t_hat))*control_points(target_rows(2),col_xy(1)) + (t_hat.^2)*control_points(target_rows(3),col_xy(1));
%     y = ((1-t_hat).^2)*control_points(target_rows(1),col_xy(2)) + 2*(t_hat.*(1-t_hat))*control_points(target_rows(2),col_xy(2)) + (t_hat.^2)*control_points(target_rows(3),col_xy(2));
%     xdot = 2*(1-t_hat)*(control_points(target_rows(2),col_xy(1))-control_points(target_rows(1),col_xy(1))) + 2*t_hat*(control_points(target_rows(3),col_xy(1))-control_points(target_rows(2),col_xy(1)));
%     ydot = 2*(1-t_hat)*(control_points(target_rows(2),col_xy(2))-control_points(target_rows(1),col_xy(2))) + 2*t_hat*(control_points(target_rows(3),col_xy(2))-control_points(target_rows(2),col_xy(2)));
%     xdotdot = 2*(control_points(target_rows(3),col_xy(1)) - 2*control_points(target_rows(2),col_xy(1)) + control_points(target_rows(1),col_xy(1)))*ones(size(t_hat));
%     ydotdot = 2*(control_points(target_rows(3),col_xy(2)) - 2*control_points(target_rows(2),col_xy(2)) + control_points(target_rows(1),col_xy(2)))*ones(size(t_hat));
%     curv = abs(xdot.*ydotdot - ydot.*xdotdot)./((xdot.^2 + ydot.^2).^1.5); %curvature along the bezier curve
%     arcvel = curv.^(-2/3);
    
    
    pos = ((1-t)^2)*control_points(target_rows(1),col_xy) + 2*(t*(1-t))*control_points(target_rows(2),col_xy) + (t^2)*control_points(target_rows(3),col_xy);
elseif (length(target_rows) == 4)
    
%     %reshape t from purely linear to some nicely shaped speed following the
%     %2/3 power law?
%     x = ((1-t_hat).^3)*control_points(target_rows(1),col_xy(1)) + 3*(t_hat.*(1-t_hat).^2)*control_points(target_rows(2),col_xy(1)) + 3*((1-t_hat).*(t_hat.^2))*control_points(target_rows(3),col_xy(1)) + (t_hat.^3)*control_points(target_rows(4),col_xy(1));
%     y = ((1-t_hat).^3)*control_points(target_rows(1),col_xy(2)) + 3*(t_hat.*(1-t_hat).^2)*control_points(target_rows(2),col_xy(2)) + 3*((1-t_hat).*(t_hat.^2))*control_points(target_rows(3),col_xy(2)) + (t_hat.^3)*control_points(target_rows(4),col_xy(2));
%     xdot = 3*((1-t_hat).^2)*(control_points(target_rows(2),col_xy(1))-control_points(target_rows(1),col_xy(1))) + 6*((1-t_hat).*t_hat)*(control_points(target_rows(3),col_xy(1))-control_points(target_rows(2),col_xy(1))) + 3*(t_hat.^2)*(control_points(target_rows(4),col_xy(1))-control_points(target_rows(3),col_xy(1)));
%     ydot = 3*((1-t_hat).^2)*(control_points(target_rows(2),col_xy(2))-control_points(target_rows(1),col_xy(2))) + 6*((1-t_hat).*t_hat)*(control_points(target_rows(3),col_xy(2))-control_points(target_rows(2),col_xy(2))) + 3*(t_hat.^2)*(control_points(target_rows(4),col_xy(2))-control_points(target_rows(3),col_xy(2)));
%     xdotdot = 6*(1-t_hat)*(control_points(target_rows(3),col_xy(1))-2*control_points(target_rows(2),col_xy(1))+control_points(target_rows(1),col_xy(1))) + 6*(t_hat)*(control_points(target_rows(4),col_xy(1))-2*control_points(target_rows(3),col_xy(1))+control_points(target_rows(2),col_xy(1)));
%     ydotdot = 6*(1-t_hat)*(control_points(target_rows(3),col_xy(2))-2*control_points(target_rows(2),col_xy(2))+control_points(target_rows(1),col_xy(2))) + 6*(t_hat)*(control_points(target_rows(4),col_xy(2))-2*control_points(target_rows(3),col_xy(2))+control_points(target_rows(2),col_xy(2)));
%     curv = abs(xdot.*ydotdot - ydot.*xdotdot)./((xdot.^2 + ydot.^2).^1.5); %curvature along the bezier curve
%     arcvel = curv.^(-2/3);

    
    pos = ((1-t)^3)*control_points(target_rows(1),col_xy) + 3*(t*(1-t)^2)*control_points(target_rows(2),col_xy) + 3*((t^2)*(1-t))*control_points(target_rows(3),col_xy) + (t^3)*control_points(target_rows(4),col_xy);
elseif (length(target_rows) == 2)

    %t = t-sin(2*pi*t)/(2*pi);  %use the bell-shaped velocity profile from the trajectory controller
    pos = (1-t)*control_points(target_rows(1),col_xy) + (t)*control_points(target_rows(2),col_xy);
else %length == 1
    
    pos = control_points(target_rows(1),col_xy);
    
end

pos = pos/100;
pos(1) = pos(1)+offsetX;
pos(2) = pos(2)+offsetY;

VCODE_mod(3) = pos(1); %convert to meters
VCODE_mod(4) = pos(2); %convert to meters

== matlab function Imitation_Task_Multi_withSound_withGrid/Subsystem/MATLAB Function ==
  data: pos input; VCODE_MOD output; VCODE input
function VCODE_MOD = fcn(pos,VCODE)
%#codegen

VCODE_MOD = VCODE;

VCODE_MOD(3) = pos(1);
VCODE_MOD(4) = pos(2);

== matlab function Imitation_Task_Multi_withSound_withGrid/Subsystem1/MATLAB Function ==
  data: VCODE input; VCODES_GRID output size=[25 70]; StartTgtVCODE input
function VCODES_GRID  = fcn(VCODE,StartTgtVCODE)
%#codegen

%we will tile the space between (+x/-x, +y/0) at regular intervals

xmax = VCODE(3);
ymax = VCODE(4);

%xs = linspace(-xmax,xmax,Nx);
%ys = linspace(0,ymax,Ny);
xs = zeros(5,1);  %we will set the grid to always be 5 by 5 since Simulink doesn't like variable-lenth variables
ys = zeros(5,1);

startX = StartTgtVCODE(3);
startY = StartTgtVCODE(4);

xmax = abs(xmax-startX);  %get the offset relative to the start target
ymax = abs(ymax-startY);

for a = 1:5

    
    xs(a) = -xmax + (xmax*2)/4*(a-1);
    ys(a) = 0 + (ymax)/4*(a-1);
end

[gridX,gridY] = meshgrid(xs,ys);
grid = [reshape(gridX,[],1),reshape(gridY,[],1)];

%VCODE(1) = VCODE(1)+ 100;  %mark as a background target

%we will initialize this to be 30; we won't allow any more points than
%this!
VCODES_GRID = zeros(25,70);

%VCODES_GRID = repmat(VCODE,size(grid,1),1);

for a = 1:min(size(grid,1),25)
    VCODES_GRID(a,:) = VCODE;
    VCODES_GRID(a,3) = grid(a,1)+startX;
    VCODES_GRID(a,4) = grid(a,2)+startY;
    VCODES_GRID(a,8) = a+50;  %set the ID
end

pos = VCODES_GRID(:,3:4);
gridpos = reshape(pos',[],1);
